simulink model "model"  (R2014a)
settings: Solver=ode4  StartTime=0.0  StopTime=40  FixedStep=0.01  RelTol=1e-3
undefined symbols (not defined in the file or in its folder): K, martwa_strefa, T
settings Model: CovSFcnEnable=on  Creator=Piotr  LastModifiedBy=Cula
settings OptimizationCC: SimCompilerOptimization=off
settings DebuggingCC: UnderspecifiedInitializationDetection=Classic  FrameProcessingCompatibilityMsg=error
settings RTWCC: RTWCompilerOptimization=off

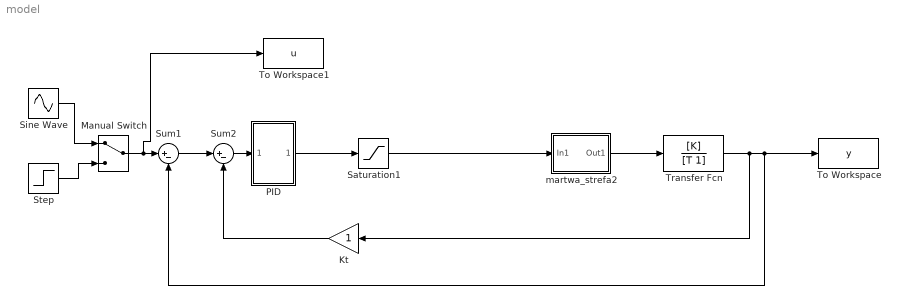
== system model ==
  Kt : Gain
  Manual Switch : ManualSwitch
  PID : Subsystem
  Saturation1 : Saturate  UpperLimit=1  LowerLimit=-1
  Sine Wave : Sin  SampleTime=0
  Step : Step  After=10  SampleTime=0
  Sum1 : Sum  Inputs=|+-
  Sum2 : Sum  Inputs=|+-
  To Workspace : ToWorkspace  VariableName=y  SaveFormat=Structure With Time  SampleTime=-1
  To Workspace1 : ToWorkspace  VariableName=u  SaveFormat=Structure With Time  SampleTime=-1
  Transfer Fcn : TransferFcn  Numerator=[K]  Denominator=[T 1]
  martwa_strefa2 : Subsystem
  wires:
  Transfer Fcn/1 -> Kt/1, To Workspace/1, Sum1/2
  Sine Wave/1 -> Manual Switch/1
  Step/1 -> Manual Switch/2
  PID/1(Out1) -> Saturation1/1
  Kt/1 -> Sum2/2
  Sum2/1 -> PID/1(In1)
  Sum1/1 -> Sum2/1
  martwa_strefa2/1(Out1) -> Transfer Fcn/1
  Manual Switch/1 -> To Workspace1/1, Sum1/1
  Saturation1/1 -> martwa_strefa2/1(In1)

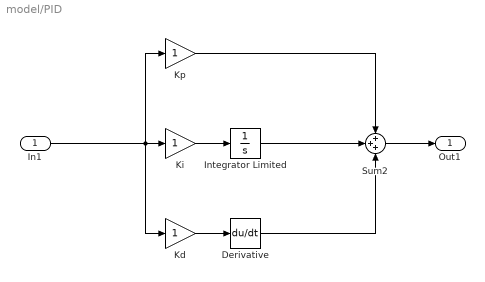
== system model/PID ==
  In1 : Inport
  Derivative : Derivative
  Integrator Limited : Integrator  LimitOutput=on  UpperSaturationLimit=1  LowerSaturationLimit=-1
  Kd : Gain
  Ki : Gain
  Kp : Gain
  Sum2 : Sum  Inputs=+++
  Out1 : Outport
  wires:
  Kp/1 -> Sum2/1
  Ki/1 -> Integrator Limited/1
  Sum2/1 -> Out1/1
  Kd/1 -> Derivative/1
  In1/1 -> Kp/1, Kd/1, Ki/1
  Derivative/1 -> Sum2/3
  Integrator Limited/1 -> Sum2/2

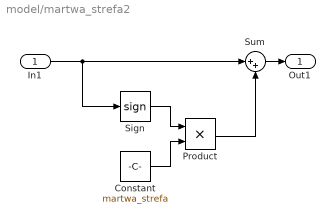
== system model/martwa_strefa2 ==
  In1 : Inport
  Constant : Constant  Value=martwa_strefa
  Product : Product
  Sign : Signum
  Sum : Sum  Inputs=|++
  Out1 : Outport
  wires:
  In1/1 -> Sum/1, Sign/1
  Product/1 -> Sum/2
  Sign/1 -> Product/1
  Constant/1 -> Product/2
  Sum/1 -> Out1/1
